simulink model "all_module"  (R2023a)
settings: Solver=VariableStepAuto  StartTime=0.0  StopTime=0.1  RelTol=1e-3
libraries: spsMosfetLib x12, powerlib_extras x11, spsVoltageMeasurementLib x9, spsSeriesRLCBranchLib x7, spsACVoltageSourceLib x4, spspowerguiLib x4, spsCurrentMeasurementLib x3, spsIGBTLib x2
settings Model: Creator=Huang  LastModifiedBy=Huang

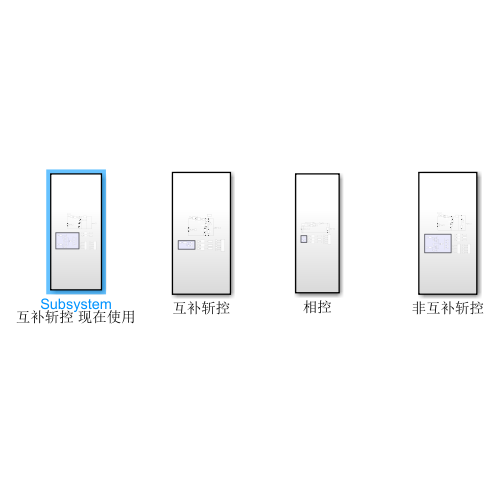
[thumbnail: Simulink's stored preview of the top-level diagram]
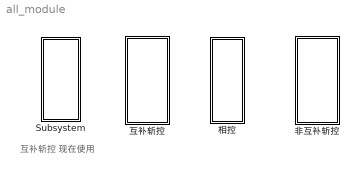
== system all_module ==
  note: 互补斩控 现在使用
  Subsystem : Subsystem
  互补斩控 : Subsystem
  相控 : Subsystem
  非互补斩控 : Subsystem

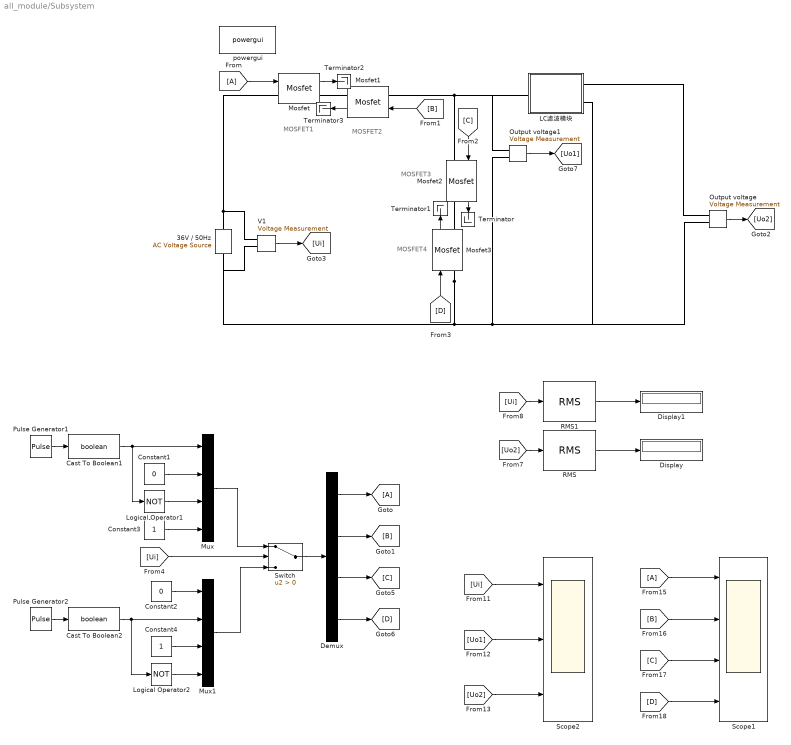
== system all_module/Subsystem ==
  note: MOSFET1
  note: MOSFET2
  note: MOSFET3
  note: MOSFET4
  36V / 50Hz : spsACVoltageSourceLib/AC Voltage Source  Amplitude=36*sqrt(2)  Phase=0  Frequency=50  SampleTime=0  Measurements=None  BusType=swing  Pref=10e3  Qref=0  Qmin=-inf  Qmax=+inf
  Cast To Boolean1 : DataTypeConversion  OutDataTypeStr=boolean  SaturateOnIntegerOverflow=off  RndMeth=Floor
  Cast To Boolean2 : DataTypeConversion  OutDataTypeStr=boolean  SaturateOnIntegerOverflow=off  RndMeth=Floor
  Constant1 : Constant  Value=0  OutDataTypeStr=boolean
  Constant2 : Constant  Value=0  OutDataTypeStr=boolean
  Constant3 : Constant  OutDataTypeStr=boolean
  Constant4 : Constant  OutDataTypeStr=boolean
  Demux : Demux
  Display : Display
  Display1 : Display
  From : From
  From15 : From
  Goto : Goto
  LC滤波模块 : Subsystem
  Logical Operator1 : Logic  Operator=NOT  AllPortsSameDT=off  OutDataTypeStr=boolean
  Logical Operator2 : Logic  Operator=NOT  AllPortsSameDT=off  OutDataTypeStr=boolean
  Mosfet{,1..3} (4 alike) : spsMosfetLib/Mosfet  Ron=0.1  Lon=0  Rd=0.01  Vfd=0  IC=0  Rs=1e5  Cs=inf  Measurements=on
  Mux : Mux
  Mux1 : Mux
  Output voltage : spsVoltageMeasurementLib/Voltage Measurement  PhasorSimulation=off  OutputType=Complex  PSBequivalent=0
  Output voltage1 : spsVoltageMeasurementLib/Voltage Measurement  PhasorSimulation=off  OutputType=Complex  PSBequivalent=0
  Pulse Generator1 : DiscretePulseGenerator  PulseType=Time based  Period=1/20e3  PulseWidth=98
  Pulse Generator2 : DiscretePulseGenerator  PulseType=Time based  Period=1/20e3  PulseWidth=98
  RMS : powerlib_extras/Measurements/RMS  f1=50
  RMS1 : powerlib_extras/Measurements/RMS  f1=50
  Scope1 : Scope  NumInputPorts=4
  Scope2 : Scope  NumInputPorts=3
  Switch : Switch  Criteria=u2 > Threshold  SaturateOnIntegerOverflow=off  InputSameDT=off
  Terminator{,1..3} (4 alike) : Terminator
  V1 : spsVoltageMeasurementLib/Voltage Measurement  PhasorSimulation=off  OutputType=Complex  PSBequivalent=0
  powergui : spspowerguiLib/powergui  Priority=1  SimulationMode=Discrete  SampleTime=1e-6  frequency=60  Iterations=50  frequencyindice=0  Pbase=100e6  ErrMax=1e-4  UnitsV=kV  UnitsW=MW  buscounter=0  FunctionMessages=off  echomessages=off  EnableUseOfTLC=off  CurrentSourceSwitches=off  DisableSnubberDevices=off  DisableRonSwitches=off  DisableVfSwitches=off  DisplayEquations=off  AutomaticDiscreteSolvers=off  SolverType=Tustin/Backward Euler (TBE)  Interpol=off  ExternalGateDelay=off  methode=off  Ts=100  x0status=blocks  SPID=on  SwTol=0  HookPort=off  NonlinearTolerance=1e-4  nMaxIteration=100  ContinueOnMaxIteration=off  RestoreLinks=warning  ResistiveCurrentMeasurement=off  Frange=[0:2:500]  Ylog=off  Xlog=on  ShowGrid=off  save=off  variable=ZData  structure=0  ZoomFFT=off  StartTime=0.0  cycles=1  DisplayStyle=1  fundamental=60  FreqAxis=off  MaxFrequency=1000  frequencyindicesteady=1  RmsSteady=1  display=off
  wires:
  Cast To Boolean1/1 -> Mux/1, Logical Operator1/1
  [C] -> Scope1/3
  Pulse Generator2/1 -> Cast To Boolean2/1
  Demux/2 -> [B]
  RMS1/1 -> Display1/1
  Mux/1 -> Switch/1
  Mux1/1 -> Switch/3
  From15/1 -> Scope1/1
  V1/1 -> [Ui]
  [Ui] -> Switch/2
  Mosfet3/1 -> Terminator1/1
  [Uo2] -> Scope2/3
  Output voltage/1 -> [Uo2]
  Mosfet/1 -> Terminator2/1
  Logical Operator1/1 -> Mux/3
  [B] -> Scope1/2
  Logical Operator2/1 -> Mux1/4
  [D] -> Scope1/4
  Mosfet2/1 -> Terminator/1
  [Uo1] -> Scope2/2
  Cast To Boolean2/1 -> Logical Operator2/1, Mux1/2
  Pulse Generator1/1 -> Cast To Boolean1/1
  Demux/1 -> Goto/1
  Demux/4 -> [D]
  [Ui] -> RMS1/1
  Demux/3 -> [C]
  Constant2/1 -> Mux1/1
  Switch/1 -> Demux/1
  Mosfet1/1 -> Terminator3/1
  [Ui] -> Scope2/1
  Constant1/1 -> Mux/2
  RMS/1 -> Display/1
  [Uo2] -> RMS/1
  Constant3/1 -> Mux/4
  Constant4/1 -> Mux1/3
  From/1 -> Mosfet/1
  [B] -> Mosfet1/1
  [C] -> Mosfet2/1
  [D] -> Mosfet3/1
  Output voltage1/1 -> [Uo1]
  connections:
  Mosfet1/RConn1 -- Mosfet/RConn1
  Mosfet1/LConn1 -- Output voltage1/LConn1 -- LC滤波模块/LConn1 -- Mosfet2/LConn1
  Mosfet3/LConn1 -- Output voltage1/LConn2 -- LC滤波模块/RConn2 -- Output voltage/LConn2 -- V1/LConn2 -- 36V / 50Hz/LConn1
  V1/LConn1 -- Mosfet/LConn1 -- 36V / 50Hz/RConn1
  Mosfet3/RConn1 -- Mosfet2/RConn1
  LC滤波模块/RConn1 -- Output voltage/LConn1

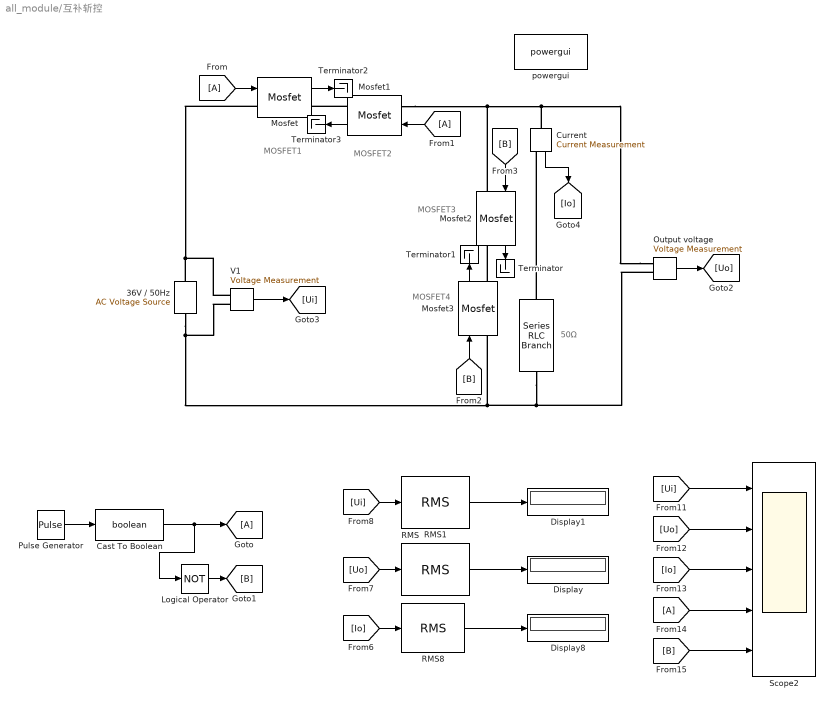
== system all_module/互补斩控 ==
  note: 50Ω
  note: MOSFET3
  note: MOSFET4
  note: MOSFET1
  note: MOSFET2
  " " : spsSeriesRLCBranchLib/Series RLC Branch  LConnTagsString=__new0  RConnTagsString=__new0  BranchType=R  Resistance=50  Inductance=0.00045  SetiL0=off  InitialCurrent=0  Capacitance=0.001  Setx0=off  InitialVoltage=0  Measurements=Branch voltage and current
  36V / 50Hz : spsACVoltageSourceLib/AC Voltage Source  Amplitude=36*sqrt(2)  Phase=0  Frequency=50  SampleTime=0  Measurements=None  BusType=swing  Pref=10e3  Qref=0  Qmin=-inf  Qmax=+inf
  Cast To Boolean : DataTypeConversion  OutDataTypeStr=boolean  SaturateOnIntegerOverflow=off  RndMeth=Floor
  "Current " : spsCurrentMeasurementLib/Current Measurement  PhasorSimulation=off  OutputType=Complex  PSBequivalent=0
  Display : Display
  Display1 : Display
  Display8 : Display
  From : From
  From1 : From
  From14 : From
  Goto : Goto
  Logical Operator : Logic  Operator=NOT  AllPortsSameDT=off  OutDataTypeStr=boolean
  Mosfet{,1..3} (4 alike) : spsMosfetLib/Mosfet  Ron=0.1  Lon=0  Rd=0.01  Vfd=0  IC=0  Rs=1e5  Cs=inf  Measurements=on
  Output voltage : spsVoltageMeasurementLib/Voltage Measurement  PhasorSimulation=off  OutputType=Complex  PSBequivalent=0
  Pulse Generator : DiscretePulseGenerator  PulseType=Time based  Period=1/20e3  PulseWidth=50
  RMS : powerlib_extras/Measurements/RMS  f1=50
  RMS1 : powerlib_extras/Measurements/RMS  f1=50
  RMS8 : powerlib_extras/Measurements/RMS  f1=50
  Scope2 : Scope  NumInputPorts=5
  Terminator{,1..3} (4 alike) : Terminator
  V1 : spsVoltageMeasurementLib/Voltage Measurement  PhasorSimulation=off  OutputType=Complex  PSBequivalent=0
  powergui : spspowerguiLib/powergui  Priority=1  SimulationMode=Discrete  SampleTime=1e-6  frequency=60  Iterations=50  frequencyindice=0  Pbase=100e6  ErrMax=1e-4  UnitsV=kV  UnitsW=MW  buscounter=0  FunctionMessages=off  echomessages=off  EnableUseOfTLC=off  CurrentSourceSwitches=off  DisableSnubberDevices=off  DisableRonSwitches=off  DisableVfSwitches=off  DisplayEquations=off  AutomaticDiscreteSolvers=off  SolverType=Tustin/Backward Euler (TBE)  Interpol=off  ExternalGateDelay=off  methode=off  Ts=100  x0status=blocks  SPID=on  SwTol=0  HookPort=off  NonlinearTolerance=1e-4  nMaxIteration=100  ContinueOnMaxIteration=off  RestoreLinks=warning  ResistiveCurrentMeasurement=off  Frange=[0:2:500]  Ylog=off  Xlog=on  ShowGrid=off  save=off  variable=ZData  structure=0  ZoomFFT=off  StartTime=0.0  cycles=1  DisplayStyle=1  fundamental=60  FreqAxis=off  MaxFrequency=1000  frequencyindicesteady=1  RmsSteady=1  display=off
  wires:
  "Current "/1 -> [Io]
  Cast To Boolean/1 -> Goto/1, Logical Operator/1
  From/1 -> Mosfet/1
  From1/1 -> Mosfet1/1
  V1/1 -> [Ui]
  Output voltage/1 -> [Uo]
  [B] -> Mosfet2/1
  Pulse Generator/1 -> Cast To Boolean/1
  Mosfet3/1 -> Terminator1/1
  Logical Operator/1 -> [B]
  [B] -> Mosfet3/1
  Mosfet/1 -> Terminator2/1
  Mosfet2/1 -> Terminator/1
  Mosfet1/1 -> Terminator3/1
  RMS1/1 -> Display1/1
  [Ui] -> RMS1/1
  [Uo] -> RMS/1
  [B] -> Scope2/5
  [Ui] -> Scope2/1
  [Uo] -> Scope2/2
  From14/1 -> Scope2/4
  RMS8/1 -> Display8/1
  [Io] -> Scope2/3
  RMS/1 -> Display/1
  [Io] -> RMS8/1
  connections:
  Mosfet3/LConn1 -- " "/RConn1 -- Output voltage/LConn2 -- 36V / 50Hz/LConn1 -- V1/LConn2
  V1/LConn1 -- 36V / 50Hz/RConn1 -- Mosfet/LConn1
  Output voltage/LConn1 -- Mosfet2/LConn1 -- Mosfet1/LConn1 -- "Current "/LConn1
  " "/LConn1 -- "Current "/RConn1
  Mosfet3/RConn1 -- Mosfet2/RConn1
  Mosfet1/RConn1 -- Mosfet/RConn1

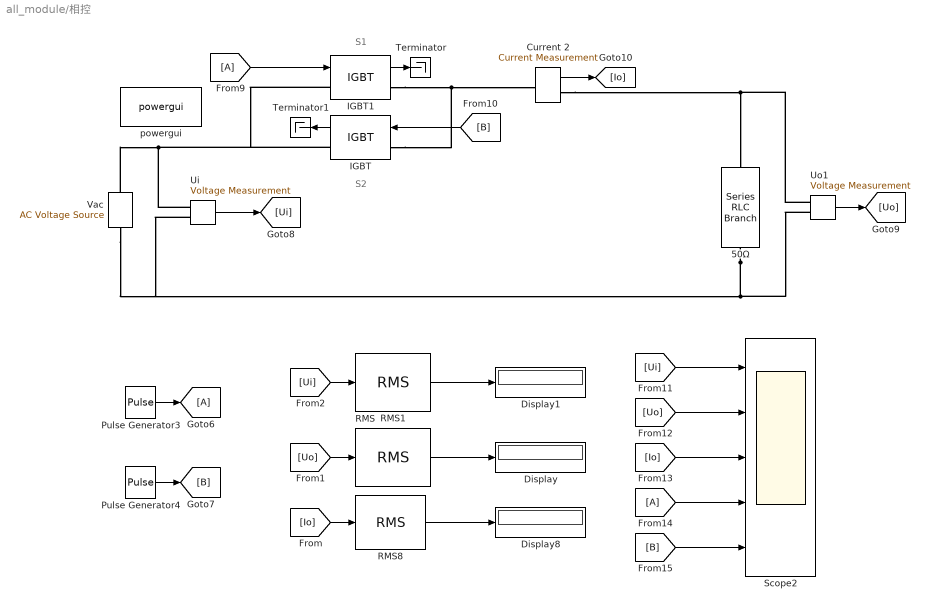
== system all_module/相控 ==
  note: S2
  note: S1
  50Ω : spsSeriesRLCBranchLib/Series RLC Branch  LConnTagsString=__new0  RConnTagsString=__new0  BranchType=R  Resistance=50  Inductance=1  SetiL0=off  InitialCurrent=0  Capacitance=1e-6  Setx0=off  InitialVoltage=0  Measurements=None
  Current 2 : spsCurrentMeasurementLib/Current Measurement  PhasorSimulation=off  OutputType=Complex  PSBequivalent=0
  Display : Display
  Display1 : Display
  Display8 : Display
  From14 : From
  From9 : From
  Goto6 : Goto
  IGBT : spsIGBTLib/IGBT  Ron=0.001  Lon=0  Vf=1  Tf=1e-6  Tt=2e-6  IC=0  Rs=1e5  Cs=inf  Measurements=on
  IGBT1 : spsIGBTLib/IGBT  Ron=0.001  Lon=0  Vf=1  Tf=1e-6  Tt=2e-6  IC=0  Rs=1e5  Cs=inf  Measurements=on
  Pulse Generator3 : DiscretePulseGenerator  PulseType=Time based  Period=1/50  PulseWidth=30  PhaseDelay=(30/180)/50
  Pulse Generator4 : DiscretePulseGenerator  PulseType=Time based  Period=1/50  PulseWidth=30  PhaseDelay=(120/180)/50
  RMS : powerlib_extras/Measurements/RMS  f1=50
  RMS1 : powerlib_extras/Measurements/RMS  f1=50
  RMS8 : powerlib_extras/Measurements/RMS  f1=50
  Scope2 : Scope  NumInputPorts=5
  Terminator : Terminator
  Terminator1 : Terminator
  Ui : spsVoltageMeasurementLib/Voltage Measurement  PhasorSimulation=off  OutputType=Complex  PSBequivalent=0
  Uo1 : spsVoltageMeasurementLib/Voltage Measurement  PhasorSimulation=off  OutputType=Complex  PSBequivalent=0
  Vac : spsACVoltageSourceLib/AC Voltage Source  Amplitude=36*sqrt(2)  Phase=0  Frequency=50  SampleTime=0  Measurements=None  BusType=swing  Pref=10e3  Qref=0  Qmin=-inf  Qmax=+inf
  powergui : spspowerguiLib/powergui  Priority=1  SimulationMode=Discrete  SampleTime=1e-5  frequency=60  Iterations=50  frequencyindice=50  Pbase=100e6  ErrMax=1e-4  UnitsV=kV  UnitsW=MW  buscounter=0  FunctionMessages=off  echomessages=off  EnableUseOfTLC=off  CurrentSourceSwitches=off  DisableSnubberDevices=off  DisableRonSwitches=off  DisableVfSwitches=off  DisplayEquations=off  AutomaticDiscreteSolvers=off  SolverType=Tustin/Backward Euler (TBE)  Interpol=off  ExternalGateDelay=off  methode=off  Ts=100  x0status=blocks  SPID=on  SwTol=0  HookPort=off  NonlinearTolerance=0  nMaxIteration=15  ContinueOnMaxIteration=off  RestoreLinks=warning  ResistiveCurrentMeasurement=off  Frange=[0:2:500]  Ylog=off  Xlog=on  ShowGrid=off  save=off  variable=ZData  structure=0  ZoomFFT=off  StartTime=0.0  cycles=1  DisplayStyle=1  fundamental=60  FreqAxis=off  MaxFrequency=1000  frequencyindicesteady=1  RmsSteady=1  display=off
  wires:
  [Io] -> Scope2/3
  RMS8/1 -> Display8/1
  From9/1 -> IGBT1/1
  [B] -> Scope2/5
  Ui/1 -> [Ui]
  Current 2/1 -> [Io]
  IGBT1/1 -> Terminator/1
  Pulse Generator3/1 -> Goto6/1
  From14/1 -> Scope2/4
  Pulse Generator4/1 -> [B]
  [Ui] -> Scope2/1
  [Uo] -> Scope2/2
  [B] -> IGBT/1
  IGBT/1 -> Terminator1/1
  [Io] -> RMS8/1
  RMS/1 -> Display/1
  Uo1/1 -> [Uo]
  [Uo] -> RMS/1
  [Ui] -> RMS1/1
  RMS1/1 -> Display1/1
  connections:
  IGBT1/RConn1 -- Current 2/LConn1 -- IGBT/LConn1
  Ui/LConn1 -- Vac/RConn1 -- IGBT1/LConn1 -- IGBT/RConn1
  50Ω/RConn1 -- Uo1/LConn2 -- Vac/LConn1 -- Ui/LConn2
  Uo1/LConn1 -- 50Ω/LConn1 -- Current 2/RConn1

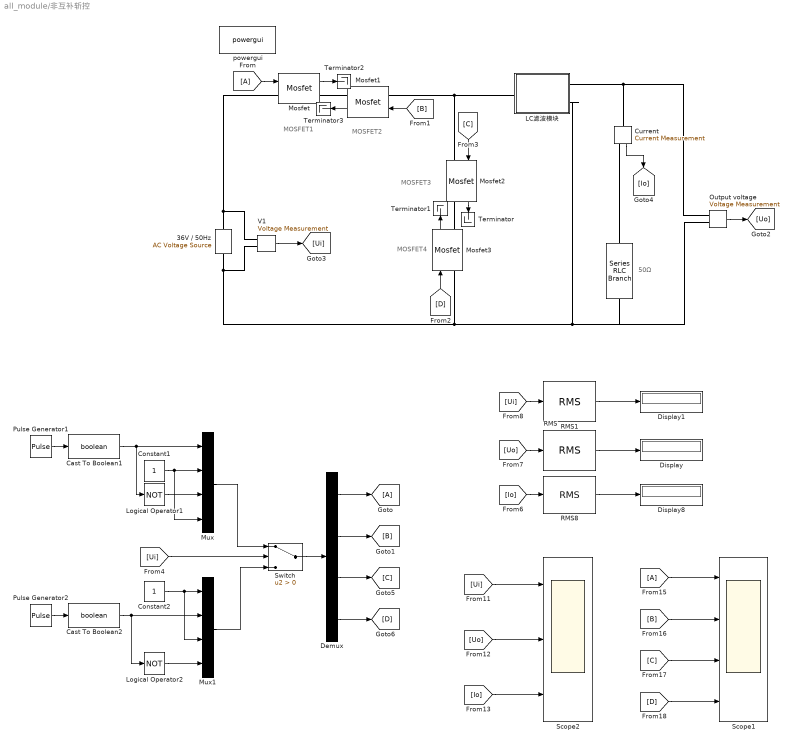
== system all_module/非互补斩控 ==
  note: MOSFET3
  note: MOSFET1
  note: 50Ω
  note: MOSFET2
  note: MOSFET4
  " " : spsSeriesRLCBranchLib/Series RLC Branch  LConnTagsString=__new0  RConnTagsString=__new0  BranchType=R  Resistance=50  Inductance=0.00045  SetiL0=off  InitialCurrent=0  Capacitance=0.001  Setx0=off  InitialVoltage=0  Measurements=Branch voltage and current
  36V / 50Hz : spsACVoltageSourceLib/AC Voltage Source  Amplitude=36*sqrt(2)  Phase=0  Frequency=50  SampleTime=0  Measurements=None  BusType=swing  Pref=10e3  Qref=0  Qmin=-inf  Qmax=+inf
  Cast To Boolean1 : DataTypeConversion  OutDataTypeStr=boolean  SaturateOnIntegerOverflow=off  RndMeth=Floor
  Cast To Boolean2 : DataTypeConversion  OutDataTypeStr=boolean  SaturateOnIntegerOverflow=off  RndMeth=Floor
  Constant1 : Constant  OutDataTypeStr=boolean
  Constant2 : Constant  OutDataTypeStr=boolean
  "Current " : spsCurrentMeasurementLib/Current Measurement  PhasorSimulation=off  OutputType=Complex  PSBequivalent=0
  Demux : Demux
  Display : Display
  Display1 : Display
  Display8 : Display
  From : From
  From15 : From
  Goto : Goto
  LC滤波模块 : Subsystem
  Logical Operator1 : Logic  Operator=NOT  AllPortsSameDT=off  OutDataTypeStr=boolean
  Logical Operator2 : Logic  Operator=NOT  AllPortsSameDT=off  OutDataTypeStr=boolean
  Mosfet{,1..3} (4 alike) : spsMosfetLib/Mosfet  Ron=0.1  Lon=0  Rd=0.01  Vfd=0  IC=0  Rs=1e5  Cs=inf  Measurements=on
  Mux : Mux
  Mux1 : Mux
  Output voltage : spsVoltageMeasurementLib/Voltage Measurement  PhasorSimulation=off  OutputType=Complex  PSBequivalent=0
  Pulse Generator1 : DiscretePulseGenerator  PulseType=Time based  Period=1/20e3  PulseWidth=50
  Pulse Generator2 : DiscretePulseGenerator  PulseType=Time based  Period=1/20e3  PulseWidth=50
  RMS : powerlib_extras/Measurements/RMS  f1=50
  RMS1 : powerlib_extras/Measurements/RMS  f1=50
  RMS8 : powerlib_extras/Measurements/RMS  f1=50
  Scope1 : Scope  NumInputPorts=4
  Scope2 : Scope  NumInputPorts=3
  Switch : Switch  Criteria=u2 > Threshold  SaturateOnIntegerOverflow=off  InputSameDT=off
  Terminator{,1..3} (4 alike) : Terminator
  V1 : spsVoltageMeasurementLib/Voltage Measurement  PhasorSimulation=off  OutputType=Complex  PSBequivalent=0
  powergui : spspowerguiLib/powergui  Priority=1  SimulationMode=Discrete  SampleTime=1e-6  frequency=60  Iterations=50  frequencyindice=0  Pbase=100e6  ErrMax=1e-4  UnitsV=kV  UnitsW=MW  buscounter=0  FunctionMessages=off  echomessages=off  EnableUseOfTLC=off  CurrentSourceSwitches=off  DisableSnubberDevices=off  DisableRonSwitches=off  DisableVfSwitches=off  DisplayEquations=off  AutomaticDiscreteSolvers=off  SolverType=Tustin/Backward Euler (TBE)  Interpol=off  ExternalGateDelay=off  methode=off  Ts=100  x0status=blocks  SPID=on  SwTol=0  HookPort=off  NonlinearTolerance=1e-4  nMaxIteration=100  ContinueOnMaxIteration=off  RestoreLinks=warning  ResistiveCurrentMeasurement=off  Frange=[0:2:500]  Ylog=off  Xlog=on  ShowGrid=off  save=off  variable=ZData  structure=0  ZoomFFT=off  StartTime=0.0  cycles=1  DisplayStyle=1  fundamental=60  FreqAxis=off  MaxFrequency=1000  frequencyindicesteady=1  RmsSteady=1  display=off
  wires:
  Constant1/1 -> Mux/2, Mux/4
  Mux/1 -> Switch/1
  Cast To Boolean2/1 -> Logical Operator2/1, Mux1/2
  Logical Operator1/1 -> Mux/3
  Pulse Generator2/1 -> Cast To Boolean2/1
  Logical Operator2/1 -> Mux1/4
  Cast To Boolean1/1 -> Logical Operator1/1, Mux/1
  Switch/1 -> Demux/1
  Pulse Generator1/1 -> Cast To Boolean1/1
  Constant2/1 -> Mux1/3, Mux1/1
  RMS/1 -> Display/1
  RMS8/1 -> Display8/1
  [Ui] -> Scope2/1
  "Current "/1 -> [Io]
  Mosfet2/1 -> Terminator/1
  [Uo] -> RMS/1
  RMS1/1 -> Display1/1
  [Ui] -> RMS1/1
  Mosfet/1 -> Terminator2/1
  Mosfet1/1 -> Terminator3/1
  From/1 -> Mosfet/1
  [C] -> Mosfet2/1
  [D] -> Mosfet3/1
  V1/1 -> [Ui]
  [Io] -> RMS8/1
  Mosfet3/1 -> Terminator1/1
  Output voltage/1 -> [Uo]
  [Io] -> Scope2/3
  [Uo] -> Scope2/2
  [B] -> Mosfet1/1
  Mux1/1 -> Switch/3
  [Ui] -> Switch/2
  [C] -> Scope1/3
  [B] -> Scope1/2
  [D] -> Scope1/4
  From15/1 -> Scope1/1
  Demux/1 -> Goto/1
  Demux/4 -> [D]
  Demux/3 -> [C]
  Demux/2 -> [B]
  connections:
  "Current "/LConn1 -- LC滤波模块/RConn1 -- Output voltage/LConn1
  V1/LConn2 -- 36V / 50Hz/LConn1 -- LC滤波模块/RConn2 -- " "/RConn1 -- Output voltage/LConn2 -- Mosfet3/LConn1
  Mosfet/LConn1 -- 36V / 50Hz/RConn1 -- V1/LConn1
  " "/LConn1 -- "Current "/RConn1
  Mosfet1/RConn1 -- Mosfet/RConn1
  Mosfet3/RConn1 -- Mosfet2/RConn1
  Mosfet1/LConn1 -- Mosfet2/LConn1 -- LC滤波模块/LConn1

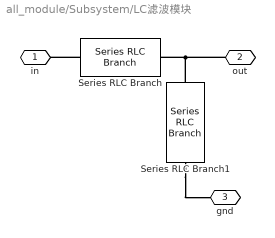
== system all_module/Subsystem/LC滤波模块 ==
  Series RLC Branch : spsSeriesRLCBranchLib/Series RLC Branch  LConnTagsString=__new0  RConnTagsString=__new0  BranchType=L  Resistance=1  Inductance=2.2e-6  SetiL0=off  InitialCurrent=0  Capacitance=1e-6  Setx0=off  InitialVoltage=0  Measurements=None
  Series RLC Branch1 : spsSeriesRLCBranchLib/Series RLC Branch  LConnTagsString=__new0  RConnTagsString=__new0  BranchType=C  Resistance=1  Inductance=1e-3  SetiL0=off  InitialCurrent=0  Capacitance=4.7e-6  Setx0=off  InitialVoltage=0  Measurements=None
  in : PMIOPort  Side=Left
  out : PMIOPort  Port=2  Side=Right
  gnd : PMIOPort  Port=3  Side=Right
  connections:
  Series RLC Branch1/RConn1 -- gnd/RConn1
  Series RLC Branch/LConn1 -- in/RConn1
  Series RLC Branch1/LConn1 -- out/RConn1 -- Series RLC Branch/RConn1

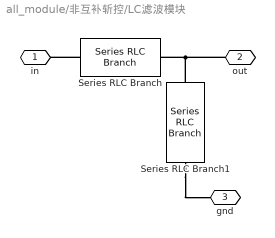
== system all_module/非互补斩控/LC滤波模块 ==
  Series RLC Branch : spsSeriesRLCBranchLib/Series RLC Branch  LConnTagsString=__new0  RConnTagsString=__new0  BranchType=L  Resistance=1  Inductance=1e-3  SetiL0=off  InitialCurrent=0  Capacitance=1e-6  Setx0=off  InitialVoltage=0  Measurements=None
  Series RLC Branch1 : spsSeriesRLCBranchLib/Series RLC Branch  LConnTagsString=__new0  RConnTagsString=__new0  BranchType=C  Resistance=1  Inductance=1e-3  SetiL0=off  InitialCurrent=0  Capacitance=1e-6  Setx0=off  InitialVoltage=0  Measurements=None
  in : PMIOPort  Side=Left
  out : PMIOPort  Port=2  Side=Right
  gnd : PMIOPort  Port=3  Side=Right
  connections:
  Series RLC Branch1/RConn1 -- gnd/RConn1
  Series RLC Branch/LConn1 -- in/RConn1
  Series RLC Branch1/LConn1 -- out/RConn1 -- Series RLC Branch/RConn1
